simulink model "DDCU_wxt_v02_forA_LabviewV02"  (R2014a)
settings: Solver=FixedStepDiscrete  StartTime=0.0  StopTime=50  FixedStep=0.0005  RelTol=1e-3
InitFcn:
  | Veh_Par_wxt
values from neighbouring files (symbols this model uses):
  ag_thr = 0.4*g    (= 3.924)    [Veh_Par_wxt.m]
  B = 2.25    [Veh_Par_wxt.m]
  bra_pre_em = 12    [Veh_Par_wxt.m]
  bra_pre_gz2 = 12/3    (= 4)    [Veh_Par_wxt.m]
  bra_pre_gz34 = 12/3    (= 4)    [Veh_Par_wxt.m]
  bra_pre_yd = 12/2    (= 6)    [Veh_Par_wxt.m]
  brakepre_dem_data = [0 1 2 3 4 5 6 7 8 9 10 11 12]    [Veh_Par_wxt.m]
  brakeTrq_dem_data = [0 218.198 436.396 654.594 872.792 1090.99 1309.188 1527.386 1745.584 1963.782 2181.98 2400.178 2618.376]    [Veh_Par_wxt.m]
  bratrq_max = 4*2618.376    (= 10473.504)    [Veh_Par_wxt.m]
  eff_tran = 0.75    [Veh_Par_wxt.m]
  G = Mass*g    (= 36297)    [Veh_Par_wxt.m]
  kd1 = 1    [Veh_Par_wxt.m]
  kd2 = 1    [Veh_Par_wxt.m]
  kd3 = 1    [Veh_Par_wxt.m]
  ki1 = 1    [Veh_Par_wxt.m]
  ki2 = 1    [Veh_Par_wxt.m]
  ki3 = 1    [Veh_Par_wxt.m]
  kp1 = 1    [Veh_Par_wxt.m]
  kp2 = 1    [Veh_Par_wxt.m]
  kp3 = 1    [Veh_Par_wxt.m]
  L = 3.12    [Veh_Par_wxt.m]
  premax = 12    [Veh_Par_wxt.m]
  Radius = 0.20    (= 0.2)    [Veh_Par_wxt.m]
  s_opt_yi_add = 0.05    [Veh_Par_wxt.m]
  s_opt_zhuan_add = 0.05    [Veh_Par_wxt.m]
  spd_map_mot = [0 100 200 300 360 400 500 600 700 800 900]*tras_ratio    [Veh_Par_wxt.m]
  spdmax = 900*tras_ratio    (= 5580)    [Veh_Par_wxt.m]
  speed_thr_park = 5/3.6/Radius*30/pi    (= 66.3145596216)    [Veh_Par_wxt.m]
  tras_ratio = 6.2    [Veh_Par_wxt.m]
  trq_map_mot = [1200 1200 1200 1200 1200 1080 864 720 617 540 480]/tras_ratio    [Veh_Par_wxt.m]
  trqmax = 80    [Veh_Par_wxt.m]
  v_thr1_b = 5    [Veh_Par_wxt.m]
  v_thr2_b = 20    [Veh_Par_wxt.m]
  v_thr_park = 5    [Veh_Par_wxt.m]
undefined symbols (not defined in the file or in its folder): DiscIntNeverNeededParam
libraries: simulink x231, ec5744lib x19
(part 4 of 16)

== system DDCU_wxt_v02_forA_LabviewV02/Data_Input/MCU1_VCU1/MCU1_VCU1 ==
  input : Inport
  Enable : EnablePort
  Demux : Demux  Outputs=8
  M1Current_Ad : Sum
  M1Current_Convert : DataTypeConversion  OutDataTypeStr=uint32
  M1Current_F : Gain  Gain=0.5
  M1Current_L : simulink/Logic and Bit Operations/Bitwise Operator  logicop=AND  UseBitMask=on  BitMask=65520  BitMaskRealWorld=Stored Integer
  M1Current_O : Constant  Value=-600  OutDataTypeStr=single
  M1Current_S : ArithShift  BitShiftNumber=4
  M1Current_Sub : Subsystem
  M1Current_sat : Saturate  UpperLimit=1447.5  LowerLimit=-600
  M1Currentcv : DataTypeConversion
  M1Currentinput3_Ad : Sum
  M1Currentinput3_C : Constant  Value=256
  M1Currentinput3_P : Product
  M1Direction_Ad : Sum
  M1Direction_Convert : DataTypeConversion  OutDataTypeStr=uint32
  M1Direction_F : Gain
  M1Direction_L : simulink/Logic and Bit Operations/Bitwise Operator  logicop=AND  UseBitMask=on  BitMask=128  BitMaskRealWorld=Stored Integer
  M1Direction_O : Constant  Value=0  OutDataTypeStr=single
  M1Direction_S : ArithShift  BitShiftNumber=7
  M1Direction_Sub : Subsystem
  M1Direction_sat : Saturate  UpperLimit=1  LowerLimit=0
  M1Directioncv : DataTypeConversion
  M1HeartBeat_Ad : Sum
  M1HeartBeat_Convert : DataTypeConversion  OutDataTypeStr=uint32
  M1HeartBeat_F : Gain
  M1HeartBeat_L : simulink/Logic and Bit Operations/Bitwise Operator  logicop=AND  UseBitMask=on  BitMask=15  BitMaskRealWorld=Stored Integer
  M1HeartBeat_O : Constant  Value=0  OutDataTypeStr=single
  M1HeartBeat_S : ArithShift
  M1HeartBeat_Sub : Subsystem
  M1HeartBeat_sat : Saturate  UpperLimit=15  LowerLimit=0
  M1HeartBeatcv : DataTypeConversion
  M1InputVolt_Ad : Sum
  M1InputVolt_Convert : DataTypeConversion  OutDataTypeStr=uint32
  M1InputVolt_F : Gain  Gain=0.25
  M1InputVolt_L : simulink/Logic and Bit Operations/Bitwise Operator  logicop=AND  UseBitMask=on  BitMask=4095  BitMaskRealWorld=Stored Integer
  M1InputVolt_O : Constant  Value=0  OutDataTypeStr=single
  M1InputVolt_S : ArithShift
  M1InputVolt_Sub : Subsystem
  M1InputVolt_sat : Saturate  UpperLimit=1023.75  LowerLimit=0
  M1InputVoltcv : DataTypeConversion
  M1InputVoltinput8_Ad : Sum
  M1InputVoltinput8_C : Constant  Value=256
  M1InputVoltinput8_P : Product
  M1Speed_Ad : Sum
  M1Speed_Convert : DataTypeConversion  OutDataTypeStr=uint32
  M1Speed_F : Gain  Gain=5
  M1Speed_L : simulink/Logic and Bit Operations/Bitwise Operator  logicop=AND  UseBitMask=on  BitMask=65535  BitMaskRealWorld=Stored Integer
  M1Speed_O : Constant  Value=-5000  OutDataTypeStr=single
  M1Speed_S : ArithShift
  M1Speed_Sub : Subsystem
  M1Speed_sat : Saturate  UpperLimit=322675  LowerLimit=-5000
  M1Speedcv : DataTypeConversion
  M1Speedinput6_Ad : Sum
  M1Speedinput6_C : Constant  Value=256
  M1Speedinput6_P : Product
  M1State_Ad : Sum
  M1State_Convert : DataTypeConversion  OutDataTypeStr=uint32
  M1State_F : Gain
  M1State_L : simulink/Logic and Bit Operations/Bitwise Operator  logicop=AND  UseBitMask=on  BitMask=112  BitMaskRealWorld=Stored Integer
  M1State_O : Constant  Value=0  OutDataTypeStr=single
  M1State_S : ArithShift  BitShiftNumber=4
  M1State_Sub : Subsystem
  M1State_sat : Saturate  UpperLimit=7  LowerLimit=0
  M1Statecv : DataTypeConversion
  M1Torque_Ad : Sum
  M1Torque_Convert : DataTypeConversion  OutDataTypeStr=uint32
  M1Torque_F : Gain  Gain=0.25
  M1Torque_L : simulink/Logic and Bit Operations/Bitwise Operator  logicop=AND  UseBitMask=on  BitMask=4095  BitMaskRealWorld=Stored Integer
  M1Torque_O : Constant  Value=-300  OutDataTypeStr=single
  M1Torque_S : ArithShift
  M1Torque_Sub : Subsystem
  M1Torque_sat : Saturate  UpperLimit=723.75  LowerLimit=-300
  M1Torquecv : DataTypeConversion
  M1Torqueinput2_Ad : Sum
  M1Torqueinput2_C : Constant  Value=256
  M1Torqueinput2_P : Product
  M1InputVolt_Out : Outport
  M1Speed_Out : Outport  Port=2
  M1Direction_Out : Outport  Port=3
  M1State_Out : Outport  Port=4
  M1HeartBeat_Out : Outport  Port=5
  M1Current_Out : Outport  Port=6
  M1Torque_Out : Outport  Port=7
  wires:
  M1InputVolt_F/1 -> M1InputVolt_Ad/1
  M1InputVolt_O/1 -> M1InputVolt_Ad/2
  M1InputVolt_Ad/1 -> M1InputVolt_sat/1
  M1InputVolt_sat/1 -> M1InputVolt_Out/1
  Demux/8 -> M1InputVoltinput8_P/1
  M1InputVoltinput8_C/1 -> M1InputVoltinput8_P/2
  M1InputVoltinput8_P/1 -> M1InputVoltinput8_Ad/1
  Demux/7 -> M1InputVoltinput8_Ad/2
  M1InputVoltinput8_Ad/1 -> M1InputVolt_Sub/1(In1)
  M1InputVolt_Sub/1(Out1) -> M1InputVolt_Convert/1
  M1InputVolt_Convert/1 -> M1InputVolt_L/1
  M1InputVolt_L/1 -> M1InputVolt_S/1
  M1InputVolt_S/1 -> M1InputVoltcv/1
  M1InputVoltcv/1 -> M1InputVolt_F/1
  M1Speed_F/1 -> M1Speed_Ad/1
  M1Speed_O/1 -> M1Speed_Ad/2
  M1Speed_Ad/1 -> M1Speed_sat/1
  M1Speed_sat/1 -> M1Speed_Out/1
  Demux/6 -> M1Speedinput6_P/1
  M1Speedinput6_C/1 -> M1Speedinput6_P/2
  M1Speedinput6_P/1 -> M1Speedinput6_Ad/1
  Demux/5 -> M1Speedinput6_Ad/2
  M1Speedinput6_Ad/1 -> M1Speed_Sub/1(In1)
  M1Speed_Sub/1(Out1) -> M1Speed_Convert/1
  M1Speed_Convert/1 -> M1Speed_L/1
  M1Speed_L/1 -> M1Speed_S/1
  M1Speed_S/1 -> M1Speedcv/1
  M1Speedcv/1 -> M1Speed_F/1
  M1Direction_F/1 -> M1Direction_Ad/1
  M1Direction_O/1 -> M1Direction_Ad/2
  M1Direction_Ad/1 -> M1Direction_sat/1
  M1Direction_sat/1 -> M1Direction_Out/1
  Demux/4 -> M1State_Sub/1(In1), M1HeartBeat_Sub/1(In1), M1Direction_Sub/1(In1)
  M1Direction_Sub/1(Out1) -> M1Direction_Convert/1
  M1Direction_Convert/1 -> M1Direction_L/1
  M1Direction_L/1 -> M1Direction_S/1
  M1Direction_S/1 -> M1Directioncv/1
  M1Directioncv/1 -> M1Direction_F/1
  M1State_F/1 -> M1State_Ad/1
  M1State_O/1 -> M1State_Ad/2
  M1State_Ad/1 -> M1State_sat/1
  M1State_sat/1 -> M1State_Out/1
  M1State_Sub/1(Out1) -> M1State_Convert/1
  M1State_Convert/1 -> M1State_L/1
  M1State_L/1 -> M1State_S/1
  M1State_S/1 -> M1Statecv/1
  M1Statecv/1 -> M1State_F/1
  M1HeartBeat_F/1 -> M1HeartBeat_Ad/1
  M1HeartBeat_O/1 -> M1HeartBeat_Ad/2
  M1HeartBeat_Ad/1 -> M1HeartBeat_sat/1
  M1HeartBeat_sat/1 -> M1HeartBeat_Out/1
  M1HeartBeat_Sub/1(Out1) -> M1HeartBeat_Convert/1
  M1HeartBeat_Convert/1 -> M1HeartBeat_L/1
  M1HeartBeat_L/1 -> M1HeartBeat_S/1
  M1HeartBeat_S/1 -> M1HeartBeatcv/1
  M1HeartBeatcv/1 -> M1HeartBeat_F/1
  M1Current_F/1 -> M1Current_Ad/1
  M1Current_O/1 -> M1Current_Ad/2
  M1Current_Ad/1 -> M1Current_sat/1
  M1Current_sat/1 -> M1Current_Out/1
  Demux/3 -> M1Currentinput3_P/1
  M1Currentinput3_C/1 -> M1Currentinput3_P/2
  M1Currentinput3_P/1 -> M1Currentinput3_Ad/1
  Demux/2 -> M1Currentinput3_Ad/2, M1Torqueinput2_P/1
  M1Currentinput3_Ad/1 -> M1Current_Sub/1(In1)
  M1Current_Sub/1(Out1) -> M1Current_Convert/1
  M1Current_Convert/1 -> M1Current_L/1
  M1Current_L/1 -> M1Current_S/1
  M1Current_S/1 -> M1Currentcv/1
  M1Currentcv/1 -> M1Current_F/1
  M1Torque_F/1 -> M1Torque_Ad/1
  M1Torque_O/1 -> M1Torque_Ad/2
  M1Torque_Ad/1 -> M1Torque_sat/1
  M1Torque_sat/1 -> M1Torque_Out/1
  M1Torqueinput2_C/1 -> M1Torqueinput2_P/2
  M1Torqueinput2_P/1 -> M1Torqueinput2_Ad/1
  Demux/1 -> M1Torqueinput2_Ad/2
  M1Torqueinput2_Ad/1 -> M1Torque_Sub/1(In1)
  M1Torque_Sub/1(Out1) -> M1Torque_Convert/1
  M1Torque_Convert/1 -> M1Torque_L/1
  M1Torque_L/1 -> M1Torque_S/1
  M1Torque_S/1 -> M1Torquecv/1
  M1Torquecv/1 -> M1Torque_F/1
  input/1 -> Demux/1

== system DDCU_wxt_v02_forA_LabviewV02/Data_Input/MCU1_VCU2/MCU1_VCU2 ==
  input : Inport
  Enable : EnablePort
  Demux : Demux  Outputs=8
  M1FaultCode_Ad : Sum
  M1FaultCode_Convert : DataTypeConversion  OutDataTypeStr=uint32
  M1FaultCode_F : Gain
  M1FaultCode_L : simulink/Logic and Bit Operations/Bitwise Operator  logicop=AND  UseBitMask=on  BitMask=65520  BitMaskRealWorld=Stored Integer
  M1FaultCode_O : Constant  Value=0  OutDataTypeStr=single
  M1FaultCode_S : ArithShift  BitShiftNumber=4
  M1FaultCode_Sub : Subsystem
  M1FaultCode_sat : Saturate  UpperLimit=4095  LowerLimit=0
  M1FaultCodecv : DataTypeConversion
  M1FaultCodeinput8_Ad : Sum
  M1FaultCodeinput8_C : Constant  Value=256
  M1FaultCodeinput8_P : Product
  M1FaultGrade_Ad : Sum
  M1FaultGrade_Convert : DataTypeConversion  OutDataTypeStr=uint32
  M1FaultGrade_F : Gain
  M1FaultGrade_L : simulink/Logic and Bit Operations/Bitwise Operator  logicop=AND  UseBitMask=on  BitMask=15  BitMaskRealWorld=Stored Integer
  M1FaultGrade_O : Constant  Value=0  OutDataTypeStr=single
  M1FaultGrade_S : ArithShift
  M1FaultGrade_Sub : Subsystem
  M1FaultGrade_sat : Saturate  UpperLimit=15  LowerLimit=0
  M1FaultGradecv : DataTypeConversion
  M1IGBTTemp_Ad : Sum
  M1IGBTTemp_Convert : DataTypeConversion  OutDataTypeStr=uint32
  M1IGBTTemp_F : Gain
  M1IGBTTemp_L : simulink/Logic and Bit Operations/Bitwise Operator  logicop=AND  UseBitMask=on  BitMask=255  BitMaskRealWorld=Stored Integer
  M1IGBTTemp_O : Constant  Value=-50  OutDataTypeStr=single
  M1IGBTTemp_S : ArithShift
  M1IGBTTemp_Sub : Subsystem
  M1IGBTTemp_sat : Saturate  UpperLimit=205  LowerLimit=-50
  M1IGBTTempcv : DataTypeConversion
  M1Temp_Ad : Sum
  M1Temp_Convert : DataTypeConversion  OutDataTypeStr=uint32
  M1Temp_F : Gain
  M1Temp_L : simulink/Logic and Bit Operations/Bitwise Operator  logicop=AND  UseBitMask=on  BitMask=255  BitMaskRealWorld=Stored Integer
  M1Temp_O : Constant  Value=-50  OutDataTypeStr=single
  M1Temp_S : ArithShift
  M1Temp_Sub : Subsystem
  M1Temp_sat : Saturate  UpperLimit=205  LowerLimit=-50
  M1Tempcv : DataTypeConversion
  M1TqLimit_Ad : Sum
  M1TqLimit_Convert : DataTypeConversion  OutDataTypeStr=uint32
  M1TqLimit_F : Gain  Gain=0.125
  M1TqLimit_L : simulink/Logic and Bit Operations/Bitwise Operator  logicop=AND  UseBitMask=on  BitMask=65535  BitMaskRealWorld=Stored Integer
  M1TqLimit_O : Constant  Value=0  OutDataTypeStr=single
  M1TqLimit_S : ArithShift
  M1TqLimit_Sub : Subsystem
  M1TqLimit_sat : Saturate  UpperLimit=8191.875  LowerLimit=0
  M1TqLimitcv : DataTypeConversion
  M1TqLimitinput6_Ad : Sum
  M1TqLimitinput6_C : Constant  Value=256
  M1TqLimitinput6_P : Product
  M1FaultGrade_Out : Outport
  M1FaultCode_Out : Outport  Port=2
  M1TqLimit_Out : Outport  Port=3
  M1IGBTTemp_Out : Outport  Port=4
  M1Temp_Out : Outport  Port=5
  wires:
  M1FaultGrade_F/1 -> M1FaultGrade_Ad/1
  M1FaultGrade_O/1 -> M1FaultGrade_Ad/2
  M1FaultGrade_Ad/1 -> M1FaultGrade_sat/1
  M1FaultGrade_sat/1 -> M1FaultGrade_Out/1
  Demux/7 -> M1FaultGrade_Sub/1(In1), M1FaultCodeinput8_Ad/2
  M1FaultGrade_Sub/1(Out1) -> M1FaultGrade_Convert/1
  M1FaultGrade_Convert/1 -> M1FaultGrade_L/1
  M1FaultGrade_L/1 -> M1FaultGrade_S/1
  M1FaultGrade_S/1 -> M1FaultGradecv/1
  M1FaultGradecv/1 -> M1FaultGrade_F/1
  M1FaultCode_F/1 -> M1FaultCode_Ad/1
  M1FaultCode_O/1 -> M1FaultCode_Ad/2
  M1FaultCode_Ad/1 -> M1FaultCode_sat/1
  M1FaultCode_sat/1 -> M1FaultCode_Out/1
  Demux/8 -> M1FaultCodeinput8_P/1
  M1FaultCodeinput8_C/1 -> M1FaultCodeinput8_P/2
  M1FaultCodeinput8_P/1 -> M1FaultCodeinput8_Ad/1
  M1FaultCodeinput8_Ad/1 -> M1FaultCode_Sub/1(In1)
  M1FaultCode_Sub/1(Out1) -> M1FaultCode_Convert/1
  M1FaultCode_Convert/1 -> M1FaultCode_L/1
  M1FaultCode_L/1 -> M1FaultCode_S/1
  M1FaultCode_S/1 -> M1FaultCodecv/1
  M1FaultCodecv/1 -> M1FaultCode_F/1
  M1TqLimit_F/1 -> M1TqLimit_Ad/1
  M1TqLimit_O/1 -> M1TqLimit_Ad/2
  M1TqLimit_Ad/1 -> M1TqLimit_sat/1
  M1TqLimit_sat/1 -> M1TqLimit_Out/1
  Demux/6 -> M1TqLimitinput6_P/1
  M1TqLimitinput6_C/1 -> M1TqLimitinput6_P/2
  M1TqLimitinput6_P/1 -> M1TqLimitinput6_Ad/1
  Demux/5 -> M1TqLimitinput6_Ad/2
  M1TqLimitinput6_Ad/1 -> M1TqLimit_Sub/1(In1)
  M1TqLimit_Sub/1(Out1) -> M1TqLimit_Convert/1
  M1TqLimit_Convert/1 -> M1TqLimit_L/1
  M1TqLimit_L/1 -> M1TqLimit_S/1
  M1TqLimit_S/1 -> M1TqLimitcv/1
  M1TqLimitcv/1 -> M1TqLimit_F/1
  M1IGBTTemp_F/1 -> M1IGBTTemp_Ad/1
  M1IGBTTemp_O/1 -> M1IGBTTemp_Ad/2
  M1IGBTTemp_Ad/1 -> M1IGBTTemp_sat/1
  M1IGBTTemp_sat/1 -> M1IGBTTemp_Out/1
  Demux/2 -> M1IGBTTemp_Sub/1(In1)
  M1IGBTTemp_Sub/1(Out1) -> M1IGBTTemp_Convert/1
  M1IGBTTemp_Convert/1 -> M1IGBTTemp_L/1
  M1IGBTTemp_L/1 -> M1IGBTTemp_S/1
  M1IGBTTemp_S/1 -> M1IGBTTempcv/1
  M1IGBTTempcv/1 -> M1IGBTTemp_F/1
  M1Temp_F/1 -> M1Temp_Ad/1
  M1Temp_O/1 -> M1Temp_Ad/2
  M1Temp_Ad/1 -> M1Temp_sat/1
  M1Temp_sat/1 -> M1Temp_Out/1
  Demux/1 -> M1Temp_Sub/1(In1)
  M1Temp_Sub/1(Out1) -> M1Temp_Convert/1
  M1Temp_Convert/1 -> M1Temp_L/1
  M1Temp_L/1 -> M1Temp_S/1
  M1Temp_S/1 -> M1Tempcv/1
  M1Tempcv/1 -> M1Temp_F/1
  input/1 -> Demux/1

== matlab function DDCU_wxt_v02_forA_LabviewV02/MainControl/mode_control/backward/backward/Brake/HeartBeat ==
  data: life_pre input; life output
function life = fcn(life_pre)
%#codegen
life=life_pre+1;
if life>15
    life=0;
end
end

== matlab function DDCU_wxt_v02_forA_LabviewV02/MainControl/mode_control/emergency_stop/emergency_stop/HeartBeat ==
  data: life_pre input; life output
function life = fcn(life_pre)
%#codegen
life=life_pre+1;
if life>15
    life=0;
end
end

== matlab function DDCU_wxt_v02_forA_LabviewV02/MainControl/mode_control/forward/forward/Drive/驱动防滑控制TCS/直行TCS/直行/MATLAB Function4 ==
  data: trq_dem_lf input; trq_dem_lr input; trq_dem_rf input; trq_dem_rr input; bra_pre_l input; bra_pre_r input; brakepre_dem input; flag_lf input; flag_lr input; trq_out_lf output; flag_rf input; flag_rr input; trq_out_lr output; trq_out_rf output; trq_out_rr output; trq_pid_lf input; trq_pid_lr input; trq_pid_rf input; trq_pid_rr input; brapre_out_l output; brapre_out_r output; mode output
function [trq_out_lf,trq_out_lr,trq_out_rf,trq_out_rr,brapre_out_l,brapre_out_r,mode] = fcn(trq_dem_lf,trq_dem_lr,trq_dem_rf,trq_dem_rr,bra_pre_l,bra_pre_r,brakepre_dem,flag_lf,flag_lr,flag_rf,flag_rr,trq_pid_lf,trq_pid_lr,trq_pid_rf,trq_pid_rr)
%#codegen pid模块在外面做，里面进行十六种情况的判断，先看一下效果，不能再修改。
if flag_lf==0 && flag_lr==0 && flag_rf==0 && flag_rr==0 % 0电机滑转===============================================0电机滑转
    trq_out_lf=trq_dem_lf;
    trq_out_lr=trq_dem_lr;
    trq_out_rf=trq_dem_rf;
    trq_out_rr=trq_dem_rr;
    brapre_out_l=bra_pre_l+brakepre_dem;
    brapre_out_r=bra_pre_r+brakepre_dem;
    mode=1;
elseif flag_lf==1 && flag_lr==0 &&flag_rf==0 && flag_rr==0 %左前轮滑转===================================================1电机滑转
    trq_out_lf=trq_pid_lf;
    trq_out_lr=trq_dem_lr+(trq_dem_lf-trq_out_lf);
    trq_out_rf=trq_dem_rf;
    trq_out_rr=trq_dem_rr;
    brapre_out_l=bra_pre_l+brakepre_dem;
    brapre_out_r=bra_pre_r+brakepre_dem;
    mode=2;
elseif flag_lf==0 && flag_lr==1 &&flag_rf==0 && flag_rr==0 %左后轮滑转
    trq_out_lr=trq_pid_lr;
    trq_out_lf=trq_dem_lf+(trq_dem_lr-trq_out_lr);
    trq_out_rf=trq_dem_rf;
    trq_out_rr=trq_dem_rr;
    brapre_out_l=bra_pre_l+brakepre_dem;
    brapre_out_r=bra_pre_r+brakepre_dem;
    mode=3;
elseif flag_lf==0 && flag_lr==0 &&flag_rf==1 && flag_rr==0 %右前轮滑转
    trq_out_rf=trq_pid_rf;
    trq_out_rr=trq_dem_rr+(trq_dem_rf-trq_out_rf);
    trq_out_lf=trq_dem_lf;
    trq_out_lr=trq_dem_lr;
    brapre_out_l=bra_pre_l+brakepre_dem;
    brapre_out_r=bra_pre_r+brakepre_dem;
    mode=4;
elseif flag_lf==0 && flag_lr==0 &&flag_rf==0 && flag_rr==1 %右后轮滑转
    trq_out_rr=trq_pid_rr;
    trq_out_rf=trq_dem_rf+(trq_dem_rr-trq_out_rr);
    trq_out_lf=trq_dem_lf;
    trq_out_lr=trq_dem_lr;
    brapre_out_l=bra_pre_l+brakepre_dem;
    brapre_out_r=bra_pre_r+brakepre_dem;
    mode=5;
elseif flag_lf==1 && flag_lr==1 &&flag_rf==0 && flag_rr==0 %左侧两轮滑转=====================================================================2电机滑转
    trq_out_lf=trq_pid_lf;
    trq_out_lr=trq_pid_lr;
    trq_out_rf=trq_dem_rf-(trq_dem_lf+trq_dem_lr-trq_out_lf-trq_out_lr)/2;
    trq_out_rr=trq_dem_rr-(trq_dem_lf+trq_dem_lr-trq_out_lf-trq_out_lr)/2;
    brapre_out_l=bra_pre_l+brakepre_dem;
    brapre_out_r=bra_pre_r+brakepre_dem;
    mode=6;
elseif flag_lf==0 && flag_lr==0 &&flag_rf==1 && flag_rr==1 %右侧两轮滑转
    trq_out_rf=trq_pid_rf;
    trq_out_rr=trq_pid_rr;
    trq_out_lf=trq_dem_lf-(trq_dem_rf+trq_dem_rr-trq_out_rf-trq_out_rr)/2;
    trq_out_lr=trq_dem_lr-(trq_dem_rf+trq_dem_rr-trq_out_rf-trq_out_rr)/2;
    brapre_out_l=bra_pre_l+brakepre_dem;
    brapre_out_r=bra_pre_r+brakepre_dem;
    mode=7;
elseif flag_lf==1 && flag_lr==0 &&flag_rf==1 && flag_rr==0 %前轴滑转
    trq_out_lf=trq_pid_lf;
    trq_out_lr=trq_dem_lr+(trq_dem_lf-trq_out_lf);
    trq_out_rf=trq_pid_rf;
    trq_out_rr=trq_dem_rr+(trq_dem_rf-trq_out_rf);
    brapre_out_l=bra_pre_l+brakepre_dem;
    brapre_out_r=bra_pre_r+brakepre_dem;
    mode=8;
elseif flag_lf==0 && flag_lr==1 &&flag_rf==0 && flag_rr==1 %后轴滑转
    trq_out_lr=trq_pid_lr;
    trq_out_lf=trq_dem_lf+(trq_dem_lr-trq_out_lr);
    trq_out_rr=trq_pid_rr;
    trq_out_rf=trq_dem_rf+(trq_dem_rr-trq_out_rr);
    brapre_out_l=bra_pre_l+brakepre_dem;
    brapre_out_r=bra_pre_r+brakepre_dem;
    mode=9;
elseif flag_lf==1 && flag_lr==0 &&flag_rf==0 && flag_rr==1 %左前轮和右后轮滑转
    trq_out_lf=trq_pid_lf;
    trq_out_lr=trq_dem_lr+(trq_dem_lf-trq_out_lf);
    trq_out_rr=trq_pid_rr;
    trq_out_rf=trq_dem_rf+(trq_dem_rr-trq_out_rr);
    brapre_out_l=bra_pre_l+brakepre_dem;
    brapre_out_r=bra_pre_r+brakepre_dem;
    mode=10;
elseif flag_lf==0 && flag_lr==1 &&flag_rf==1 && flag_rr==0 %左后轮和右前轮滑转
    trq_out_lr=trq_pid_lr;
    trq_out_lf=trq_dem_lf+(trq_dem_lr-trq_out_lr);
    trq_out_rf=trq_pid_rf;
    trq_out_rr=trq_dem_rr+(trq_dem_rf-trq_out_rf);
    brapre_out_l=bra_pre_l+brakepre_dem;
    brapre_out_r=bra_pre_r+brakepre_dem;
    mode=11;
elseif flag_lf==1 && flag_lr==1 &&flag_rf==1 && flag_rr==0 %右后不滑转======================================================================3电机滑转
    trq_out_lf=trq_pid_lf;
    trq_out_lr=trq_pid_lr;
    trq_out_rf=trq_pid_rf;
    trq_out_rr=trq_dem_rr+(trq_dem_rf-trq_out_rf)-(trq_dem_lf+trq_dem_lr-trq_out_lf-trq_out_lr);
    brapre_out_l=bra_pre_l+brakepre_dem;
    brapre_out_r=bra_pre_r+brakepre_dem;
    mode=12;
elseif flag_lf==1 && flag_lr==1 &&flag_rf==0 && flag_rr==1 %右前不滑转
    trq_out_lf=trq_pid_lf;
    trq_out_lr=trq_pid_lr;
    trq_out_rr=trq_pid_rr;
    trq_out_rf=trq_dem_rf+(trq_dem_rr-trq_out_rr)-(trq_dem_lf+trq_dem_lr-trq_out_lf-trq_out_lr);
    brapre_out_l=bra_pre_l+brakepre_dem;
    brapre_out_r=bra_pre_r+brakepre_dem;
    mode=13;
elseif flag_lf==1 && flag_lr==0 &&flag_rf==1 && flag_rr==1 %左后不滑转
    trq_out_rf=trq_pid_rf;
    trq_out_rr=trq_pid_rr;
    trq_out_lf=trq_pid_lf;
    trq_out_lr=trq_dem_lr+(trq_dem_lf-trq_out_lf)-(trq_dem_rf+trq_dem_rr-trq_out_rf-trq_out_rr);
    brapre_out_l=bra_pre_l+brakepre_dem;
    brapre_out_r=bra_pre_r+brakepre_dem;
    mode=14;
elseif flag_lf==0 && flag_lr==1 &&flag_rf==1 && flag_rr==1 %左前不滑转
    trq_out_rf=trq_pid_rf;
    trq_out_rr=trq_pid_rr;
    trq_out_lr=trq_pid_lr;
    trq_out_lf=trq_dem_lf+(trq_dem_lr-trq_out_lr)-(trq_dem_rf+trq_dem_rr-trq_out_rf-trq_out_rr);
    brapre_out_l=bra_pre_l+brakepre_dem;
    brapre_out_r=bra_pre_r+brakepre_dem;
    mode=15;
else
    %     flag_lf==1 && flag_lr==1 &&flag_rf==1 && flag_rr==1 %4电机均滑转======================================================================4电机均滑转
    trqcha=(trq_pid_lf+trq_pid_lr)-(trq_pid_rf+trq_pid_rr);
    if trqcha>0
        trq_out_rf=trq_pid_rf;
        trq_out_rr=trq_pid_rr;
        trq_out_lf=trq_pid_lf-(trq_pid_lf/(trq_pid_lf+trq_pid_lr))*trqcha;
        trq_out_lr=trq_pid_lr-(trq_pid_lr/(trq_pid_lf+trq_pid_lr))*trqcha;
    else
        trq_out_lf=trq_pid_lf;
        trq_out_lr=trq_pid_lr;
        trq_out_rf=trq_pid_rf+(trq_pid_rf/(trq_pid_rf+trq_pid_rr))*trqcha;
        trq_out_rr=trq_pid_rr+(trq_pid_rr/(trq_pid_rf+trq_pid_rr))*trqcha;
    end
    brapre_out_l=bra_pre_l+brakepre_dem;
    brapre_out_r=bra_pre_r+brakepre_dem;
    mode=16;
end
trq_out_lf=max(0,trq_out_lf);
trq_out_lr=max(0,trq_out_lr);
trq_out_rf=max(0,trq_out_rf);
trq_out_rr=max(0,trq_out_rr);
brapre_out_l=brapre_out_l;
brapre_out_r=brapre_out_r;
end

== system DDCU_wxt_v02_forA_LabviewV02/Data_Input/MCU1_VCU3/MCU1_VCU3 ==
  input : Inport
  Enable : EnablePort
  Demux : Demux  Outputs=8
  M2Current_Ad : Sum
  M2Current_Convert : DataTypeConversion  OutDataTypeStr=uint32
  M2Current_F : Gain  Gain=0.5
  M2Current_L : simulink/Logic and Bit Operations/Bitwise Operator  logicop=AND  UseBitMask=on  BitMask=65520  BitMaskRealWorld=Stored Integer
  M2Current_O : Constant  Value=-600  OutDataTypeStr=single
  M2Current_S : ArithShift  BitShiftNumber=4
  M2Current_Sub : Subsystem
  M2Current_sat : Saturate  UpperLimit=1447.5  LowerLimit=-600
  M2Currentcv : DataTypeConversion
  M2Currentinput3_Ad : Sum
  M2Currentinput3_C : Constant  Value=256
  M2Currentinput3_P : Product
  M2Direction_Ad : Sum
  M2Direction_Convert : DataTypeConversion  OutDataTypeStr=uint32
  M2Direction_F : Gain
  M2Direction_L : simulink/Logic and Bit Operations/Bitwise Operator  logicop=AND  UseBitMask=on  BitMask=128  BitMaskRealWorld=Stored Integer
  M2Direction_O : Constant  Value=0  OutDataTypeStr=single
  M2Direction_S : ArithShift  BitShiftNumber=7
  M2Direction_Sub : Subsystem
  M2Direction_sat : Saturate  UpperLimit=1  LowerLimit=0
  M2Directioncv : DataTypeConversion
  M2HeartBeat_Ad : Sum
  M2HeartBeat_Convert : DataTypeConversion  OutDataTypeStr=uint32
  M2HeartBeat_F : Gain
  M2HeartBeat_L : simulink/Logic and Bit Operations/Bitwise Operator  logicop=AND  UseBitMask=on  BitMask=15  BitMaskRealWorld=Stored Integer
  M2HeartBeat_O : Constant  Value=0  OutDataTypeStr=single
  M2HeartBeat_S : ArithShift
  M2HeartBeat_Sub : Subsystem
  M2HeartBeat_sat : Saturate  UpperLimit=15  LowerLimit=0
  M2HeartBeatcv : DataTypeConversion
  M2InputVolt_Ad : Sum
  M2InputVolt_Convert : DataTypeConversion  OutDataTypeStr=uint32
  M2InputVolt_F : Gain  Gain=0.25
  M2InputVolt_L : simulink/Logic and Bit Operations/Bitwise Operator  logicop=AND  UseBitMask=on  BitMask=4095  BitMaskRealWorld=Stored Integer
  M2InputVolt_O : Constant  Value=0  OutDataTypeStr=single
  M2InputVolt_S : ArithShift
  M2InputVolt_Sub : Subsystem
  M2InputVolt_sat : Saturate  UpperLimit=1023.75  LowerLimit=0
  M2InputVoltcv : DataTypeConversion
  M2InputVoltinput8_Ad : Sum
  M2InputVoltinput8_C : Constant  Value=256
  M2InputVoltinput8_P : Product
  M2Speed_Ad : Sum
  M2Speed_Convert : DataTypeConversion  OutDataTypeStr=uint32
  M2Speed_F : Gain  Gain=5
  M2Speed_L : simulink/Logic and Bit Operations/Bitwise Operator  logicop=AND  UseBitMask=on  BitMask=65535  BitMaskRealWorld=Stored Integer
  M2Speed_O : Constant  Value=-5000  OutDataTypeStr=single
  M2Speed_S : ArithShift
  M2Speed_Sub : Subsystem
  M2Speed_sat : Saturate  UpperLimit=322675  LowerLimit=-5000
  M2Speedcv : DataTypeConversion
  M2Speedinput6_Ad : Sum
  M2Speedinput6_C : Constant  Value=256
  M2Speedinput6_P : Product
  M2State_Ad : Sum
  M2State_Convert : DataTypeConversion  OutDataTypeStr=uint32
  M2State_F : Gain
  M2State_L : simulink/Logic and Bit Operations/Bitwise Operator  logicop=AND  UseBitMask=on  BitMask=112  BitMaskRealWorld=Stored Integer
  M2State_O : Constant  Value=0  OutDataTypeStr=single
  M2State_S : ArithShift  BitShiftNumber=4
  M2State_Sub : Subsystem
  M2State_sat : Saturate  UpperLimit=7  LowerLimit=0
  M2Statecv : DataTypeConversion
  M2Torque_Ad : Sum
  M2Torque_Convert : DataTypeConversion  OutDataTypeStr=uint32
  M2Torque_F : Gain  Gain=0.25
  M2Torque_L : simulink/Logic and Bit Operations/Bitwise Operator  logicop=AND  UseBitMask=on  BitMask=4095  BitMaskRealWorld=Stored Integer
  M2Torque_O : Constant  Value=-300  OutDataTypeStr=single
  M2Torque_S : ArithShift
  M2Torque_Sub : Subsystem
  M2Torque_sat : Saturate  UpperLimit=723.75  LowerLimit=-300
  M2Torquecv : DataTypeConversion
  M2Torqueinput2_Ad : Sum
  M2Torqueinput2_C : Constant  Value=256
  M2Torqueinput2_P : Product
  M2InputVolt_Out : Outport
  M2Speed_Out : Outport  Port=2
  M2Direction_Out : Outport  Port=3
  M2State_Out : Outport  Port=4
  M2HeartBeat_Out : Outport  Port=5
  M2Current_Out : Outport  Port=6
  M2Torque_Out : Outport  Port=7
  wires:
  M2Torque_F/1 -> M2Torque_Ad/1
  M2Torque_O/1 -> M2Torque_Ad/2
  M2Torque_Ad/1 -> M2Torque_sat/1
  M2Torque_sat/1 -> M2Torque_Out/1
  Demux/2 -> M2Torqueinput2_P/1, M2Currentinput3_Ad/2
  M2Torqueinput2_C/1 -> M2Torqueinput2_P/2
  M2Torqueinput2_P/1 -> M2Torqueinput2_Ad/1
  Demux/1 -> M2Torqueinput2_Ad/2
  M2Torqueinput2_Ad/1 -> M2Torque_Sub/1(In1)
  M2Torque_Sub/1(Out1) -> M2Torque_Convert/1
  M2Torque_Convert/1 -> M2Torque_L/1
  M2Torque_L/1 -> M2Torque_S/1
  M2Torque_S/1 -> M2Torquecv/1
  M2Torquecv/1 -> M2Torque_F/1
  M2State_F/1 -> M2State_Ad/1
  M2State_O/1 -> M2State_Ad/2
  M2State_Ad/1 -> M2State_sat/1
  M2State_sat/1 -> M2State_Out/1
  Demux/4 -> M2HeartBeat_Sub/1(In1), M2Direction_Sub/1(In1), M2State_Sub/1(In1)
  M2State_Sub/1(Out1) -> M2State_Convert/1
  M2State_Convert/1 -> M2State_L/1
  M2State_L/1 -> M2State_S/1
  M2State_S/1 -> M2Statecv/1
  M2Statecv/1 -> M2State_F/1
  M2Speed_F/1 -> M2Speed_Ad/1
  M2Speed_O/1 -> M2Speed_Ad/2
  M2Speed_Ad/1 -> M2Speed_sat/1
  M2Speed_sat/1 -> M2Speed_Out/1
  Demux/6 -> M2Speedinput6_P/1
  M2Speedinput6_C/1 -> M2Speedinput6_P/2
  M2Speedinput6_P/1 -> M2Speedinput6_Ad/1
  Demux/5 -> M2Speedinput6_Ad/2
  M2Speedinput6_Ad/1 -> M2Speed_Sub/1(In1)
  M2Speed_Sub/1(Out1) -> M2Speed_Convert/1
  M2Speed_Convert/1 -> M2Speed_L/1
  M2Speed_L/1 -> M2Speed_S/1
  M2Speed_S/1 -> M2Speedcv/1
  M2Speedcv/1 -> M2Speed_F/1
  M2InputVolt_F/1 -> M2InputVolt_Ad/1
  M2InputVolt_O/1 -> M2InputVolt_Ad/2
  M2InputVolt_Ad/1 -> M2InputVolt_sat/1
  M2InputVolt_sat/1 -> M2InputVolt_Out/1
  Demux/8 -> M2InputVoltinput8_P/1
  M2InputVoltinput8_C/1 -> M2InputVoltinput8_P/2
  M2InputVoltinput8_P/1 -> M2InputVoltinput8_Ad/1
  Demux/7 -> M2InputVoltinput8_Ad/2
  M2InputVoltinput8_Ad/1 -> M2InputVolt_Sub/1(In1)
  M2InputVolt_Sub/1(Out1) -> M2InputVolt_Convert/1
  M2InputVolt_Convert/1 -> M2InputVolt_L/1
  M2InputVolt_L/1 -> M2InputVolt_S/1
  M2InputVolt_S/1 -> M2InputVoltcv/1
  M2InputVoltcv/1 -> M2InputVolt_F/1
  M2HeartBeat_F/1 -> M2HeartBeat_Ad/1
  M2HeartBeat_O/1 -> M2HeartBeat_Ad/2
  M2HeartBeat_Ad/1 -> M2HeartBeat_sat/1
  M2HeartBeat_sat/1 -> M2HeartBeat_Out/1
  M2HeartBeat_Sub/1(Out1) -> M2HeartBeat_Convert/1
  M2HeartBeat_Convert/1 -> M2HeartBeat_L/1
  M2HeartBeat_L/1 -> M2HeartBeat_S/1
  M2HeartBeat_S/1 -> M2HeartBeatcv/1
  M2HeartBeatcv/1 -> M2HeartBeat_F/1
  M2Direction_F/1 -> M2Direction_Ad/1
  M2Direction_O/1 -> M2Direction_Ad/2
  M2Direction_Ad/1 -> M2Direction_sat/1
  M2Direction_sat/1 -> M2Direction_Out/1
  M2Direction_Sub/1(Out1) -> M2Direction_Convert/1
  M2Direction_Convert/1 -> M2Direction_L/1
  M2Direction_L/1 -> M2Direction_S/1
  M2Direction_S/1 -> M2Directioncv/1
  M2Directioncv/1 -> M2Direction_F/1
  M2Current_F/1 -> M2Current_Ad/1
  M2Current_O/1 -> M2Current_Ad/2
  M2Current_Ad/1 -> M2Current_sat/1
  M2Current_sat/1 -> M2Current_Out/1
  Demux/3 -> M2Currentinput3_P/1
  M2Currentinput3_C/1 -> M2Currentinput3_P/2
  M2Currentinput3_P/1 -> M2Currentinput3_Ad/1
  M2Currentinput3_Ad/1 -> M2Current_Sub/1(In1)
  M2Current_Sub/1(Out1) -> M2Current_Convert/1
  M2Current_Convert/1 -> M2Current_L/1
  M2Current_L/1 -> M2Current_S/1
  M2Current_S/1 -> M2Currentcv/1
  M2Currentcv/1 -> M2Current_F/1
  input/1 -> Demux/1

== system DDCU_wxt_v02_forA_LabviewV02/Data_Input/MCU1_VCU4/MCU1_VCU4 ==
  input : Inport
  Enable : EnablePort
  Demux : Demux  Outputs=8
  M2FaultCode_Ad : Sum
  M2FaultCode_Convert : DataTypeConversion  OutDataTypeStr=uint32
  M2FaultCode_F : Gain
  M2FaultCode_L : simulink/Logic and Bit Operations/Bitwise Operator  logicop=AND  UseBitMask=on  BitMask=65520  BitMaskRealWorld=Stored Integer
  M2FaultCode_O : Constant  Value=0  OutDataTypeStr=single
  M2FaultCode_S : ArithShift  BitShiftNumber=4
  M2FaultCode_Sub : Subsystem
  M2FaultCode_sat : Saturate  UpperLimit=4095  LowerLimit=0
  M2FaultCodecv : DataTypeConversion
  M2FaultCodeinput8_Ad : Sum
  M2FaultCodeinput8_C : Constant  Value=256
  M2FaultCodeinput8_P : Product
  M2FaultGrade_Ad : Sum
  M2FaultGrade_Convert : DataTypeConversion  OutDataTypeStr=uint32
  M2FaultGrade_F : Gain
  M2FaultGrade_L : simulink/Logic and Bit Operations/Bitwise Operator  logicop=AND  UseBitMask=on  BitMask=15  BitMaskRealWorld=Stored Integer
  M2FaultGrade_O : Constant  Value=0  OutDataTypeStr=single
  M2FaultGrade_S : ArithShift
  M2FaultGrade_Sub : Subsystem
  M2FaultGrade_sat : Saturate  UpperLimit=15  LowerLimit=0
  M2FaultGradecv : DataTypeConversion
  M2IGBTTemp_Ad : Sum
  M2IGBTTemp_Convert : DataTypeConversion  OutDataTypeStr=uint32
  M2IGBTTemp_F : Gain
  M2IGBTTemp_L : simulink/Logic and Bit Operations/Bitwise Operator  logicop=AND  UseBitMask=on  BitMask=255  BitMaskRealWorld=Stored Integer
  M2IGBTTemp_O : Constant  Value=-50  OutDataTypeStr=single
  M2IGBTTemp_S : ArithShift
  M2IGBTTemp_Sub : Subsystem
  M2IGBTTemp_sat : Saturate  UpperLimit=205  LowerLimit=-50
  M2IGBTTempcv : DataTypeConversion
  M2Temp_Ad : Sum
  M2Temp_Convert : DataTypeConversion  OutDataTypeStr=uint32
  M2Temp_F : Gain
  M2Temp_L : simulink/Logic and Bit Operations/Bitwise Operator  logicop=AND  UseBitMask=on  BitMask=255  BitMaskRealWorld=Stored Integer
  M2Temp_O : Constant  Value=-50  OutDataTypeStr=single
  M2Temp_S : ArithShift
  M2Temp_Sub : Subsystem
  M2Temp_sat : Saturate  UpperLimit=205  LowerLimit=-50
  M2Tempcv : DataTypeConversion
  M2TqLimit_Ad : Sum
  M2TqLimit_Convert : DataTypeConversion  OutDataTypeStr=uint32
  M2TqLimit_F : Gain  Gain=0.125
  M2TqLimit_L : simulink/Logic and Bit Operations/Bitwise Operator  logicop=AND  UseBitMask=on  BitMask=65535  BitMaskRealWorld=Stored Integer
  M2TqLimit_O : Constant  Value=0  OutDataTypeStr=single
  M2TqLimit_S : ArithShift
  M2TqLimit_Sub : Subsystem
  M2TqLimit_sat : Saturate  UpperLimit=8191.875  LowerLimit=0
  M2TqLimitcv : DataTypeConversion
  M2TqLimitinput6_Ad : Sum
  M2TqLimitinput6_C : Constant  Value=256
  M2TqLimitinput6_P : Product
  M2FaultGrade_Out : Outport
  M2FaultCode_Out : Outport  Port=2
  M2TqLimit_Out : Outport  Port=3
  M2IGBTTemp_Out : Outport  Port=4
  M2Temp_Out : Outport  Port=5
  wires:
  M2FaultCode_F/1 -> M2FaultCode_Ad/1
  M2FaultCode_O/1 -> M2FaultCode_Ad/2
  M2FaultCode_Ad/1 -> M2FaultCode_sat/1
  M2FaultCode_sat/1 -> M2FaultCode_Out/1
  Demux/8 -> M2FaultCodeinput8_P/1
  M2FaultCodeinput8_C/1 -> M2FaultCodeinput8_P/2
  M2FaultCodeinput8_P/1 -> M2FaultCodeinput8_Ad/1
  Demux/7 -> M2FaultCodeinput8_Ad/2, M2FaultGrade_Sub/1(In1)
  M2FaultCodeinput8_Ad/1 -> M2FaultCode_Sub/1(In1)
  M2FaultCode_Sub/1(Out1) -> M2FaultCode_Convert/1
  M2FaultCode_Convert/1 -> M2FaultCode_L/1
  M2FaultCode_L/1 -> M2FaultCode_S/1
  M2FaultCode_S/1 -> M2FaultCodecv/1
  M2FaultCodecv/1 -> M2FaultCode_F/1
  M2FaultGrade_F/1 -> M2FaultGrade_Ad/1
  M2FaultGrade_O/1 -> M2FaultGrade_Ad/2
  M2FaultGrade_Ad/1 -> M2FaultGrade_sat/1
  M2FaultGrade_sat/1 -> M2FaultGrade_Out/1
  M2FaultGrade_Sub/1(Out1) -> M2FaultGrade_Convert/1
  M2FaultGrade_Convert/1 -> M2FaultGrade_L/1
  M2FaultGrade_L/1 -> M2FaultGrade_S/1
  M2FaultGrade_S/1 -> M2FaultGradecv/1
  M2FaultGradecv/1 -> M2FaultGrade_F/1
  M2TqLimit_F/1 -> M2TqLimit_Ad/1
  M2TqLimit_O/1 -> M2TqLimit_Ad/2
  M2TqLimit_Ad/1 -> M2TqLimit_sat/1
  M2TqLimit_sat/1 -> M2TqLimit_Out/1
  Demux/6 -> M2TqLimitinput6_P/1
  M2TqLimitinput6_C/1 -> M2TqLimitinput6_P/2
  M2TqLimitinput6_P/1 -> M2TqLimitinput6_Ad/1
  Demux/5 -> M2TqLimitinput6_Ad/2
  M2TqLimitinput6_Ad/1 -> M2TqLimit_Sub/1(In1)
  M2TqLimit_Sub/1(Out1) -> M2TqLimit_Convert/1
  M2TqLimit_Convert/1 -> M2TqLimit_L/1
  M2TqLimit_L/1 -> M2TqLimit_S/1
  M2TqLimit_S/1 -> M2TqLimitcv/1
  M2TqLimitcv/1 -> M2TqLimit_F/1
  M2IGBTTemp_F/1 -> M2IGBTTemp_Ad/1
  M2IGBTTemp_O/1 -> M2IGBTTemp_Ad/2
  M2IGBTTemp_Ad/1 -> M2IGBTTemp_sat/1
  M2IGBTTemp_sat/1 -> M2IGBTTemp_Out/1
  Demux/2 -> M2IGBTTemp_Sub/1(In1)
  M2IGBTTemp_Sub/1(Out1) -> M2IGBTTemp_Convert/1
  M2IGBTTemp_Convert/1 -> M2IGBTTemp_L/1
  M2IGBTTemp_L/1 -> M2IGBTTemp_S/1
  M2IGBTTemp_S/1 -> M2IGBTTempcv/1
  M2IGBTTempcv/1 -> M2IGBTTemp_F/1
  M2Temp_F/1 -> M2Temp_Ad/1
  M2Temp_O/1 -> M2Temp_Ad/2
  M2Temp_Ad/1 -> M2Temp_sat/1
  M2Temp_sat/1 -> M2Temp_Out/1
  Demux/1 -> M2Temp_Sub/1(In1)
  M2Temp_Sub/1(Out1) -> M2Temp_Convert/1
  M2Temp_Convert/1 -> M2Temp_L/1
  M2Temp_L/1 -> M2Temp_S/1
  M2Temp_S/1 -> M2Tempcv/1
  M2Tempcv/1 -> M2Temp_F/1
  input/1 -> Demux/1

== system DDCU_wxt_v02_forA_LabviewV02/Data_Input/MCU2_VCU1/MCU2_VCU1 ==
  input : Inport
  Enable : EnablePort
  Demux : Demux  Outputs=8
  M3Current_Ad : Sum
  M3Current_Convert : DataTypeConversion  OutDataTypeStr=uint32
  M3Current_F : Gain  Gain=0.5
  M3Current_L : simulink/Logic and Bit Operations/Bitwise Operator  logicop=AND  UseBitMask=on  BitMask=65520  BitMaskRealWorld=Stored Integer
  M3Current_O : Constant  Value=-600  OutDataTypeStr=single
  M3Current_S : ArithShift  BitShiftNumber=4
  M3Current_Sub : Subsystem
  M3Current_sat : Saturate  UpperLimit=1447.5  LowerLimit=-600
  M3Currentcv : DataTypeConversion
  M3Currentinput3_Ad : Sum
  M3Currentinput3_C : Constant  Value=256
  M3Currentinput3_P : Product
  M3Direction_Ad : Sum
  M3Direction_Convert : DataTypeConversion  OutDataTypeStr=uint32
  M3Direction_F : Gain
  M3Direction_L : simulink/Logic and Bit Operations/Bitwise Operator  logicop=AND  UseBitMask=on  BitMask=128  BitMaskRealWorld=Stored Integer
  M3Direction_O : Constant  Value=0  OutDataTypeStr=single
  M3Direction_S : ArithShift  BitShiftNumber=7
  M3Direction_Sub : Subsystem
  M3Direction_sat : Saturate  UpperLimit=1  LowerLimit=0
  M3Directioncv : DataTypeConversion
  M3HeartBeat_Ad : Sum
  M3HeartBeat_Convert : DataTypeConversion  OutDataTypeStr=uint32
  M3HeartBeat_F : Gain
  M3HeartBeat_L : simulink/Logic and Bit Operations/Bitwise Operator  logicop=AND  UseBitMask=on  BitMask=15  BitMaskRealWorld=Stored Integer
  M3HeartBeat_O : Constant  Value=0  OutDataTypeStr=single
  M3HeartBeat_S : ArithShift
  M3HeartBeat_Sub : Subsystem
  M3HeartBeat_sat : Saturate  UpperLimit=15  LowerLimit=0
  M3HeartBeatcv : DataTypeConversion
  M3InputVolt_Ad : Sum
  M3InputVolt_Convert : DataTypeConversion  OutDataTypeStr=uint32
  M3InputVolt_F : Gain  Gain=0.25
  M3InputVolt_L : simulink/Logic and Bit Operations/Bitwise Operator  logicop=AND  UseBitMask=on  BitMask=4095  BitMaskRealWorld=Stored Integer
  M3InputVolt_O : Constant  Value=0  OutDataTypeStr=single
  M3InputVolt_S : ArithShift
  M3InputVolt_Sub : Subsystem
  M3InputVolt_sat : Saturate  UpperLimit=1023.75  LowerLimit=0
  M3InputVoltcv : DataTypeConversion
  M3InputVoltinput8_Ad : Sum
  M3InputVoltinput8_C : Constant  Value=256
  M3InputVoltinput8_P : Product
  M3Speed_Ad : Sum
  M3Speed_Convert : DataTypeConversion  OutDataTypeStr=uint32
  M3Speed_F : Gain  Gain=5
  M3Speed_L : simulink/Logic and Bit Operations/Bitwise Operator  logicop=AND  UseBitMask=on  BitMask=65535  BitMaskRealWorld=Stored Integer
  M3Speed_O : Constant  Value=-5000  OutDataTypeStr=single
  M3Speed_S : ArithShift
  M3Speed_Sub : Subsystem
  M3Speed_sat : Saturate  UpperLimit=322675  LowerLimit=-5000
  M3Speedcv : DataTypeConversion
  M3Speedinput6_Ad : Sum
  M3Speedinput6_C : Constant  Value=256
  M3Speedinput6_P : Product
  M3State_Ad : Sum
  M3State_Convert : DataTypeConversion  OutDataTypeStr=uint32
  M3State_F : Gain
  M3State_L : simulink/Logic and Bit Operations/Bitwise Operator  logicop=AND  UseBitMask=on  BitMask=112  BitMaskRealWorld=Stored Integer
  M3State_O : Constant  Value=0  OutDataTypeStr=single
  M3State_S : ArithShift  BitShiftNumber=4
  M3State_Sub : Subsystem
  M3State_sat : Saturate  UpperLimit=7  LowerLimit=0
  M3Statecv : DataTypeConversion
  M3Torque_Ad : Sum
  M3Torque_Convert : DataTypeConversion  OutDataTypeStr=uint32
  M3Torque_F : Gain  Gain=0.25
  M3Torque_L : simulink/Logic and Bit Operations/Bitwise Operator  logicop=AND  UseBitMask=on  BitMask=4095  BitMaskRealWorld=Stored Integer
  M3Torque_O : Constant  Value=-300  OutDataTypeStr=single
  M3Torque_S : ArithShift
  M3Torque_Sub : Subsystem
  M3Torque_sat : Saturate  UpperLimit=723.75  LowerLimit=-300
  M3Torquecv : DataTypeConversion
  M3Torqueinput2_Ad : Sum
  M3Torqueinput2_C : Constant  Value=256
  M3Torqueinput2_P : Product
  M3InputVolt_Out : Outport
  M3Speed_Out : Outport  Port=2
  M3Direction_Out : Outport  Port=3
  M3State_Out : Outport  Port=4
  M3HeartBeat_Out : Outport  Port=5
  M3Current_Out : Outport  Port=6
  M3Torque_Out : Outport  Port=7
  wires:
  M3InputVolt_F/1 -> M3InputVolt_Ad/1
  M3InputVolt_O/1 -> M3InputVolt_Ad/2
  M3InputVolt_Ad/1 -> M3InputVolt_sat/1
  M3InputVolt_sat/1 -> M3InputVolt_Out/1
  Demux/8 -> M3InputVoltinput8_P/1
  M3InputVoltinput8_C/1 -> M3InputVoltinput8_P/2
  M3InputVoltinput8_P/1 -> M3InputVoltinput8_Ad/1
  Demux/7 -> M3InputVoltinput8_Ad/2
  M3InputVoltinput8_Ad/1 -> M3InputVolt_Sub/1(In1)
  M3InputVolt_Sub/1(Out1) -> M3InputVolt_Convert/1
  M3InputVolt_Convert/1 -> M3InputVolt_L/1
  M3InputVolt_L/1 -> M3InputVolt_S/1
  M3InputVolt_S/1 -> M3InputVoltcv/1
  M3InputVoltcv/1 -> M3InputVolt_F/1
  M3Speed_F/1 -> M3Speed_Ad/1
  M3Speed_O/1 -> M3Speed_Ad/2
  M3Speed_Ad/1 -> M3Speed_sat/1
  M3Speed_sat/1 -> M3Speed_Out/1
  Demux/6 -> M3Speedinput6_P/1
  M3Speedinput6_C/1 -> M3Speedinput6_P/2
  M3Speedinput6_P/1 -> M3Speedinput6_Ad/1
  Demux/5 -> M3Speedinput6_Ad/2
  M3Speedinput6_Ad/1 -> M3Speed_Sub/1(In1)
  M3Speed_Sub/1(Out1) -> M3Speed_Convert/1
  M3Speed_Convert/1 -> M3Speed_L/1
  M3Speed_L/1 -> M3Speed_S/1
  M3Speed_S/1 -> M3Speedcv/1
  M3Speedcv/1 -> M3Speed_F/1
  M3Direction_F/1 -> M3Direction_Ad/1
  M3Direction_O/1 -> M3Direction_Ad/2
  M3Direction_Ad/1 -> M3Direction_sat/1
  M3Direction_sat/1 -> M3Direction_Out/1
  Demux/4 -> M3State_Sub/1(In1), M3HeartBeat_Sub/1(In1), M3Direction_Sub/1(In1)
  M3Direction_Sub/1(Out1) -> M3Direction_Convert/1
  M3Direction_Convert/1 -> M3Direction_L/1
  M3Direction_L/1 -> M3Direction_S/1
  M3Direction_S/1 -> M3Directioncv/1
  M3Directioncv/1 -> M3Direction_F/1
  M3State_F/1 -> M3State_Ad/1
  M3State_O/1 -> M3State_Ad/2
  M3State_Ad/1 -> M3State_sat/1
  M3State_sat/1 -> M3State_Out/1
  M3State_Sub/1(Out1) -> M3State_Convert/1
  M3State_Convert/1 -> M3State_L/1
  M3State_L/1 -> M3State_S/1
  M3State_S/1 -> M3Statecv/1
  M3Statecv/1 -> M3State_F/1
  M3HeartBeat_F/1 -> M3HeartBeat_Ad/1
  M3HeartBeat_O/1 -> M3HeartBeat_Ad/2
  M3HeartBeat_Ad/1 -> M3HeartBeat_sat/1
  M3HeartBeat_sat/1 -> M3HeartBeat_Out/1
  M3HeartBeat_Sub/1(Out1) -> M3HeartBeat_Convert/1
  M3HeartBeat_Convert/1 -> M3HeartBeat_L/1
  M3HeartBeat_L/1 -> M3HeartBeat_S/1
  M3HeartBeat_S/1 -> M3HeartBeatcv/1
  M3HeartBeatcv/1 -> M3HeartBeat_F/1
  M3Current_F/1 -> M3Current_Ad/1
  M3Current_O/1 -> M3Current_Ad/2
  M3Current_Ad/1 -> M3Current_sat/1
  M3Current_sat/1 -> M3Current_Out/1
  Demux/3 -> M3Currentinput3_P/1
  M3Currentinput3_C/1 -> M3Currentinput3_P/2
  M3Currentinput3_P/1 -> M3Currentinput3_Ad/1
  Demux/2 -> M3Currentinput3_Ad/2, M3Torqueinput2_P/1
  M3Currentinput3_Ad/1 -> M3Current_Sub/1(In1)
  M3Current_Sub/1(Out1) -> M3Current_Convert/1
  M3Current_Convert/1 -> M3Current_L/1
  M3Current_L/1 -> M3Current_S/1
  M3Current_S/1 -> M3Currentcv/1
  M3Currentcv/1 -> M3Current_F/1
  M3Torque_F/1 -> M3Torque_Ad/1
  M3Torque_O/1 -> M3Torque_Ad/2
  M3Torque_Ad/1 -> M3Torque_sat/1
  M3Torque_sat/1 -> M3Torque_Out/1
  M3Torqueinput2_C/1 -> M3Torqueinput2_P/2
  M3Torqueinput2_P/1 -> M3Torqueinput2_Ad/1
  Demux/1 -> M3Torqueinput2_Ad/2
  M3Torqueinput2_Ad/1 -> M3Torque_Sub/1(In1)
  M3Torque_Sub/1(Out1) -> M3Torque_Convert/1
  M3Torque_Convert/1 -> M3Torque_L/1
  M3Torque_L/1 -> M3Torque_S/1
  M3Torque_S/1 -> M3Torquecv/1
  M3Torquecv/1 -> M3Torque_F/1
  input/1 -> Demux/1

== system DDCU_wxt_v02_forA_LabviewV02/Data_Input/MCU2_VCU2/MCU2_VCU2 ==
  input : Inport
  Enable : EnablePort
  Demux : Demux  Outputs=8
  M3FaultCode_Ad : Sum
  M3FaultCode_Convert : DataTypeConversion  OutDataTypeStr=uint32
  M3FaultCode_F : Gain
  M3FaultCode_L : simulink/Logic and Bit Operations/Bitwise Operator  logicop=AND  UseBitMask=on  BitMask=65520  BitMaskRealWorld=Stored Integer
  M3FaultCode_O : Constant  Value=0  OutDataTypeStr=single
  M3FaultCode_S : ArithShift  BitShiftNumber=4
  M3FaultCode_Sub : Subsystem
  M3FaultCode_sat : Saturate  UpperLimit=4095  LowerLimit=0
  M3FaultCodecv : DataTypeConversion
  M3FaultCodeinput8_Ad : Sum
  M3FaultCodeinput8_C : Constant  Value=256
  M3FaultCodeinput8_P : Product
  M3FaultGrade_Ad : Sum
  M3FaultGrade_Convert : DataTypeConversion  OutDataTypeStr=uint32
  M3FaultGrade_F : Gain
  M3FaultGrade_L : simulink/Logic and Bit Operations/Bitwise Operator  logicop=AND  UseBitMask=on  BitMask=15  BitMaskRealWorld=Stored Integer
  M3FaultGrade_O : Constant  Value=0  OutDataTypeStr=single
  M3FaultGrade_S : ArithShift
  M3FaultGrade_Sub : Subsystem
  M3FaultGrade_sat : Saturate  UpperLimit=15  LowerLimit=0
  M3FaultGradecv : DataTypeConversion
  M3IGBTTemp_Ad : Sum
  M3IGBTTemp_Convert : DataTypeConversion  OutDataTypeStr=uint32
  M3IGBTTemp_F : Gain
  M3IGBTTemp_L : simulink/Logic and Bit Operations/Bitwise Operator  logicop=AND  UseBitMask=on  BitMask=255  BitMaskRealWorld=Stored Integer
  M3IGBTTemp_O : Constant  Value=-50  OutDataTypeStr=single
  M3IGBTTemp_S : ArithShift
  M3IGBTTemp_Sub : Subsystem
  M3IGBTTemp_sat : Saturate  UpperLimit=205  LowerLimit=-50
  M3IGBTTempcv : DataTypeConversion
  M3Temp_Ad : Sum
  M3Temp_Convert : DataTypeConversion  OutDataTypeStr=uint32
  M3Temp_F : Gain
  M3Temp_L : simulink/Logic and Bit Operations/Bitwise Operator  logicop=AND  UseBitMask=on  BitMask=255  BitMaskRealWorld=Stored Integer
  M3Temp_O : Constant  Value=-50  OutDataTypeStr=single
  M3Temp_S : ArithShift
  M3Temp_Sub : Subsystem
  M3Temp_sat : Saturate  UpperLimit=205  LowerLimit=-50
  M3Tempcv : DataTypeConversion
  M3TqLimit_Ad : Sum
  M3TqLimit_Convert : DataTypeConversion  OutDataTypeStr=uint32
  M3TqLimit_F : Gain  Gain=0.125
  M3TqLimit_L : simulink/Logic and Bit Operations/Bitwise Operator  logicop=AND  UseBitMask=on  BitMask=65535  BitMaskRealWorld=Stored Integer
  M3TqLimit_O : Constant  Value=0  OutDataTypeStr=single
  M3TqLimit_S : ArithShift
  M3TqLimit_Sub : Subsystem
  M3TqLimit_sat : Saturate  UpperLimit=8191.875  LowerLimit=0
  M3TqLimitcv : DataTypeConversion
  M3TqLimitinput6_Ad : Sum
  M3TqLimitinput6_C : Constant  Value=256
  M3TqLimitinput6_P : Product
  M3FaultGrade_Out : Outport
  M3FaultCode_Out : Outport  Port=2
  M3TqLimit_Out : Outport  Port=3
  M3IGBTTemp_Out : Outport  Port=4
  M3Temp_Out : Outport  Port=5
  wires:
  M3FaultCode_F/1 -> M3FaultCode_Ad/1
  M3FaultCode_O/1 -> M3FaultCode_Ad/2
  M3FaultCode_Ad/1 -> M3FaultCode_sat/1
  M3FaultCode_sat/1 -> M3FaultCode_Out/1
  Demux/8 -> M3FaultCodeinput8_P/1
  M3FaultCodeinput8_C/1 -> M3FaultCodeinput8_P/2
  M3FaultCodeinput8_P/1 -> M3FaultCodeinput8_Ad/1
  Demux/7 -> M3FaultCodeinput8_Ad/2, M3FaultGrade_Sub/1(In1)
  M3FaultCodeinput8_Ad/1 -> M3FaultCode_Sub/1(In1)
  M3FaultCode_Sub/1(Out1) -> M3FaultCode_Convert/1
  M3FaultCode_Convert/1 -> M3FaultCode_L/1
  M3FaultCode_L/1 -> M3FaultCode_S/1
  M3FaultCode_S/1 -> M3FaultCodecv/1
  M3FaultCodecv/1 -> M3FaultCode_F/1
  M3FaultGrade_F/1 -> M3FaultGrade_Ad/1
  M3FaultGrade_O/1 -> M3FaultGrade_Ad/2
  M3FaultGrade_Ad/1 -> M3FaultGrade_sat/1
  M3FaultGrade_sat/1 -> M3FaultGrade_Out/1
  M3FaultGrade_Sub/1(Out1) -> M3FaultGrade_Convert/1
  M3FaultGrade_Convert/1 -> M3FaultGrade_L/1
  M3FaultGrade_L/1 -> M3FaultGrade_S/1
  M3FaultGrade_S/1 -> M3FaultGradecv/1
  M3FaultGradecv/1 -> M3FaultGrade_F/1
  M3TqLimit_F/1 -> M3TqLimit_Ad/1
  M3TqLimit_O/1 -> M3TqLimit_Ad/2
  M3TqLimit_Ad/1 -> M3TqLimit_sat/1
  M3TqLimit_sat/1 -> M3TqLimit_Out/1
  Demux/6 -> M3TqLimitinput6_P/1
  M3TqLimitinput6_C/1 -> M3TqLimitinput6_P/2
  M3TqLimitinput6_P/1 -> M3TqLimitinput6_Ad/1
  Demux/5 -> M3TqLimitinput6_Ad/2
  M3TqLimitinput6_Ad/1 -> M3TqLimit_Sub/1(In1)
  M3TqLimit_Sub/1(Out1) -> M3TqLimit_Convert/1
  M3TqLimit_Convert/1 -> M3TqLimit_L/1
  M3TqLimit_L/1 -> M3TqLimit_S/1
  M3TqLimit_S/1 -> M3TqLimitcv/1
  M3TqLimitcv/1 -> M3TqLimit_F/1
  M3IGBTTemp_F/1 -> M3IGBTTemp_Ad/1
  M3IGBTTemp_O/1 -> M3IGBTTemp_Ad/2
  M3IGBTTemp_Ad/1 -> M3IGBTTemp_sat/1
  M3IGBTTemp_sat/1 -> M3IGBTTemp_Out/1
  Demux/2 -> M3IGBTTemp_Sub/1(In1)
  M3IGBTTemp_Sub/1(Out1) -> M3IGBTTemp_Convert/1
  M3IGBTTemp_Convert/1 -> M3IGBTTemp_L/1
  M3IGBTTemp_L/1 -> M3IGBTTemp_S/1
  M3IGBTTemp_S/1 -> M3IGBTTempcv/1
  M3IGBTTempcv/1 -> M3IGBTTemp_F/1
  M3Temp_F/1 -> M3Temp_Ad/1
  M3Temp_O/1 -> M3Temp_Ad/2
  M3Temp_Ad/1 -> M3Temp_sat/1
  M3Temp_sat/1 -> M3Temp_Out/1
  Demux/1 -> M3Temp_Sub/1(In1)
  M3Temp_Sub/1(Out1) -> M3Temp_Convert/1
  M3Temp_Convert/1 -> M3Temp_L/1
  M3Temp_L/1 -> M3Temp_S/1
  M3Temp_S/1 -> M3Tempcv/1
  M3Tempcv/1 -> M3Temp_F/1
  input/1 -> Demux/1
